simulink model "cardio_v4"  (Simulink 7.4)
settings: Solver=ode45  StartTime=0.0  StopTime=10  FixedStep=0.1  RelTol=1e-3
undefined symbols (not defined in the file): ln
(part 2 of 2)

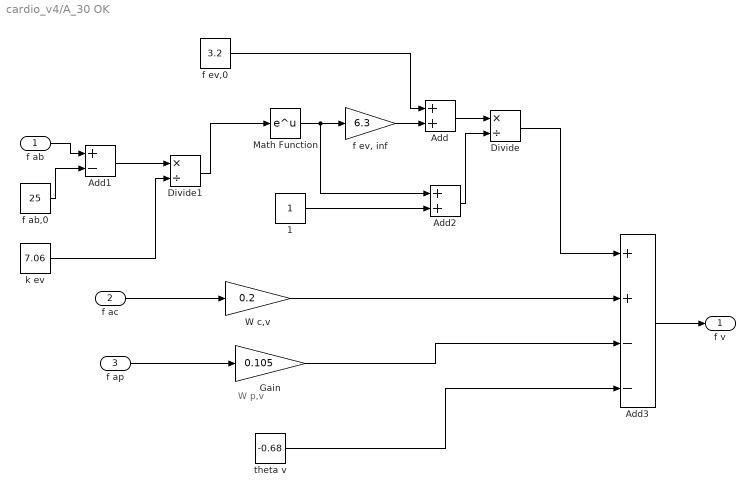
== system cardio_v4/A_30 OK ==
  note: W p,v
  f ab : Inport  OutDataType=sfix(16)  OutScaling=2^0
  f ac : Inport  Port=2  OutDataType=sfix(16)  OutScaling=2^0
  f ap : Inport  Port=3  OutDataType=sfix(16)  OutScaling=2^0
  1 : Constant  OutDataType=sfix(16)  OutScaling=2^0
  Add : Sum  OutDataType=sfix(16)  OutScaling=2^-10
  Add1 : Sum  Inputs=+-  OutDataType=sfix(16)  OutScaling=2^-10
  Add2 : Sum  OutDataType=sfix(16)  OutScaling=2^-10
  Add3 : Sum  Inputs=++--  OutDataType=sfix(16)  OutScaling=2^-10
  Divide : Product  Inputs=*/  OutDataType=sfix(16)  OutScaling=2^-10
  Divide1 : Product  Inputs=*/  OutDataType=sfix(16)  OutScaling=2^-10
  Gain : Gain  Gain=0.105  ParameterDataType=sfix(16)  ParameterScaling=2^0  OutDataType=sfix(16)  OutScaling=2^0
  Math Function : Math  OutDataType=sfix(16)  OutScaling=2^0  SaturateOnIntegerOverflow=on
  W c,v : Gain  Gain=0.2  ParameterDataType=sfix(16)  ParameterScaling=2^0  OutDataType=sfix(16)  OutScaling=2^0
  f ab,0 : Constant  Value=25  OutDataType=sfix(16)  OutScaling=2^0
  "f ev, inf" : Gain  Gain=6.3  ParameterDataType=sfix(16)  ParameterScaling=2^0  OutDataType=sfix(16)  OutScaling=2^0
  f ev,0 : Constant  Value=3.2  OutDataType=sfix(16)  OutScaling=2^0
  k ev : Constant  Value=7.06  OutDataType=sfix(16)  OutScaling=2^0
  theta v : Constant  Value=-0.68  OutDataType=sfix(16)  OutScaling=2^0
  f v : Outport  OutDataType=sfix(16)  OutScaling=2^0
  wires:
  theta v/1 -> Add3/4
  Gain/1 -> Add3/3
  f ap/1 -> Gain/1
  f ac/1 -> W c,v/1
  W c,v/1 -> Add3/2
  Add3/1 -> f v/1
  Divide/1 -> Add3/1
  1/1 -> Add2/2
  Add2/1 -> Divide/2
  k ev/1 -> Divide1/2
  Divide1/1 -> Math Function/1
  Add1/1 -> Divide1/1
  f ab,0/1 -> Add1/2
  f ab/1 -> Add1/1
  Math Function/1 -> Add2/1, "f ev, inf"/1
  "f ev, inf"/1 -> Add/2
  f ev,0/1 -> Add/1
  Add/1 -> Divide/1

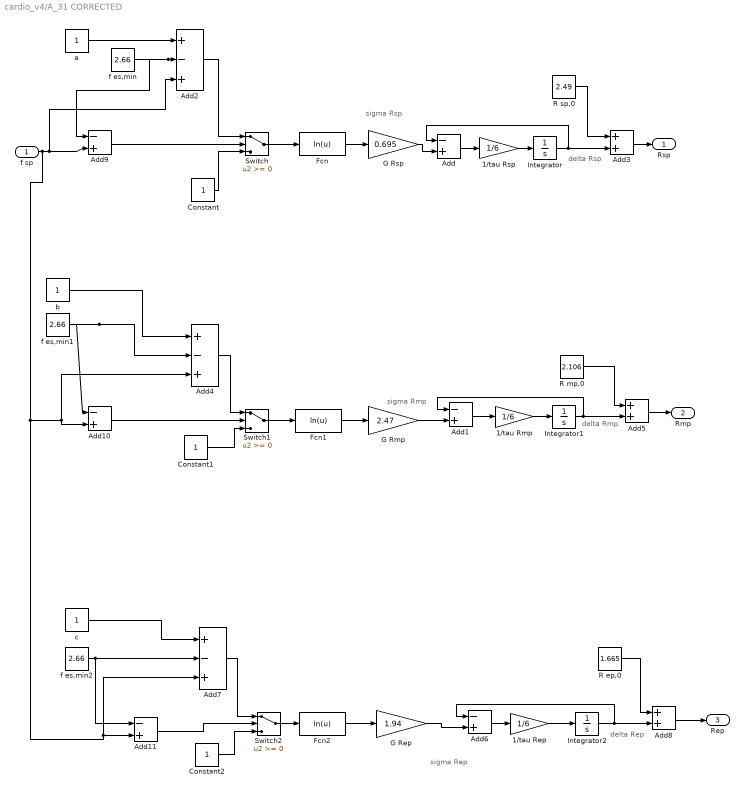
== system cardio_v4/A_31 CORRECTED ==
  note: sigma Rep
  note: delta Rep
  note: delta Rmp
  note: sigma Rmp
  note: delta Rsp
  note: sigma Rsp
  f sp : Inport  OutDataType=sfix(16)  OutScaling=2^0
  1/tau Rep : Gain  Gain=1/6  ParameterDataType=sfix(16)  ParameterScaling=2^0  OutDataType=sfix(16)  OutScaling=2^0
  1/tau Rmp : Gain  Gain=1/6  ParameterDataType=sfix(16)  ParameterScaling=2^0  OutDataType=sfix(16)  OutScaling=2^0
  1/tau Rsp : Gain  Gain=1/6  ParameterDataType=sfix(16)  ParameterScaling=2^0  OutDataType=sfix(16)  OutScaling=2^0
  Add{,1,6,9..11} (6 alike) : Sum  Inputs=-+  OutDataType=sfix(16)  OutScaling=2^-10
  Add2 : Sum  Inputs=+-+  OutDataType=sfix(16)  OutScaling=2^-10
  Add3 : Sum  OutDataType=sfix(16)  OutScaling=2^-10
  Add4 : Sum  Inputs=+-+  OutDataType=sfix(16)  OutScaling=2^-10
  Add5 : Sum  OutDataType=sfix(16)  OutScaling=2^-10
  Add7 : Sum  Inputs=+-+  OutDataType=sfix(16)  OutScaling=2^-10
  Add8 : Sum  OutDataType=sfix(16)  OutScaling=2^-10
  Constant : Constant  OutDataType=sfix(16)  OutScaling=2^0
  Constant1 : Constant  OutDataType=sfix(16)  OutScaling=2^0
  Constant2 : Constant  OutDataType=sfix(16)  OutScaling=2^0
  Fcn : Fcn  Expr=ln(u)
  Fcn1 : Fcn  Expr=ln(u)
  Fcn2 : Fcn  Expr=ln(u)
  G Rep : Gain  Gain=1.94  ParameterDataType=sfix(16)  ParameterScaling=2^0  OutDataType=sfix(16)  OutScaling=2^0
  G Rmp : Gain  Gain=2.47  ParameterDataType=sfix(16)  ParameterScaling=2^0  OutDataType=sfix(16)  OutScaling=2^0
  G Rsp : Gain  Gain=0.695  ParameterDataType=sfix(16)  ParameterScaling=2^0  OutDataType=sfix(16)  OutScaling=2^0
  Integrator : Integrator
  Integrator1 : Integrator
  Integrator2 : Integrator
  R ep,0 : Constant  Value=1.665  OutDataType=sfix(16)  OutScaling=2^0
  R mp,0 : Constant  Value=2.106  OutDataType=sfix(16)  OutScaling=2^0
  R sp,0 : Constant  Value=2.49  OutDataType=sfix(16)  OutScaling=2^0
  Switch : Switch
  Switch1 : Switch
  Switch2 : Switch
  a : Constant  OutDataType=sfix(16)  OutScaling=2^0
  b : Constant  OutDataType=sfix(16)  OutScaling=2^0
  c : Constant  OutDataType=sfix(16)  OutScaling=2^0
  f es,min : Constant  Value=2.66  OutDataType=sfix(16)  OutScaling=2^0
  f es,min1 : Constant  Value=2.66  OutDataType=sfix(16)  OutScaling=2^0
  f es,min2 : Constant  Value=2.66  OutDataType=sfix(16)  OutScaling=2^0
  Rsp : Outport  OutDataType=sfix(16)  OutScaling=2^0
  Rmp : Outport  Port=2  OutDataType=sfix(16)  OutScaling=2^0
  Rep : Outport  Port=3  OutDataType=sfix(16)  OutScaling=2^0
  wires:
  R mp,0/1 -> Add5/1
  Add5/1 -> Rmp/1
  f es,min/1 -> Add2/2, Add9/1
  a/1 -> Add2/1
  R sp,0/1 -> Add3/1
  R ep,0/1 -> Add8/1
  Add8/1 -> Rep/1
  f es,min2/1 -> Add7/2, Add11/1
  c/1 -> Add7/1
  Fcn2/1 -> G Rep/1
  Integrator2/1 -> Add8/2, Add6/1
  Add6/1 -> 1/tau Rep/1
  1/tau Rep/1 -> Integrator2/1
  f es,min1/1 -> Add4/2, Add10/1
  b/1 -> Add4/1
  Fcn1/1 -> G Rmp/1
  Integrator1/1 -> Add5/2, Add1/1
  Add1/1 -> 1/tau Rmp/1
  1/tau Rmp/1 -> Integrator1/1
  Add3/1 -> Rsp/1
  Fcn/1 -> G Rsp/1
  f sp/1 -> Add10/2, Add4/3, Add11/2, Add7/3, Add9/2, Add2/3
  Integrator/1 -> Add3/2, Add/1
  Add/1 -> 1/tau Rsp/1
  1/tau Rsp/1 -> Integrator/1
  Constant/1 -> Switch/3
  Add9/1 -> Switch/2
  Add2/1 -> Switch/1
  Switch/1 -> Fcn/1
  G Rsp/1 -> Add/2
  Add10/1 -> Switch1/2
  Constant1/1 -> Switch1/3
  Add4/1 -> Switch1/1
  Switch1/1 -> Fcn1/1
  G Rmp/1 -> Add1/2
  Constant2/1 -> Switch2/3
  Add11/1 -> Switch2/2
  Add7/1 -> Switch2/1
  Switch2/1 -> Fcn2/1
  G Rep/1 -> Add6/2

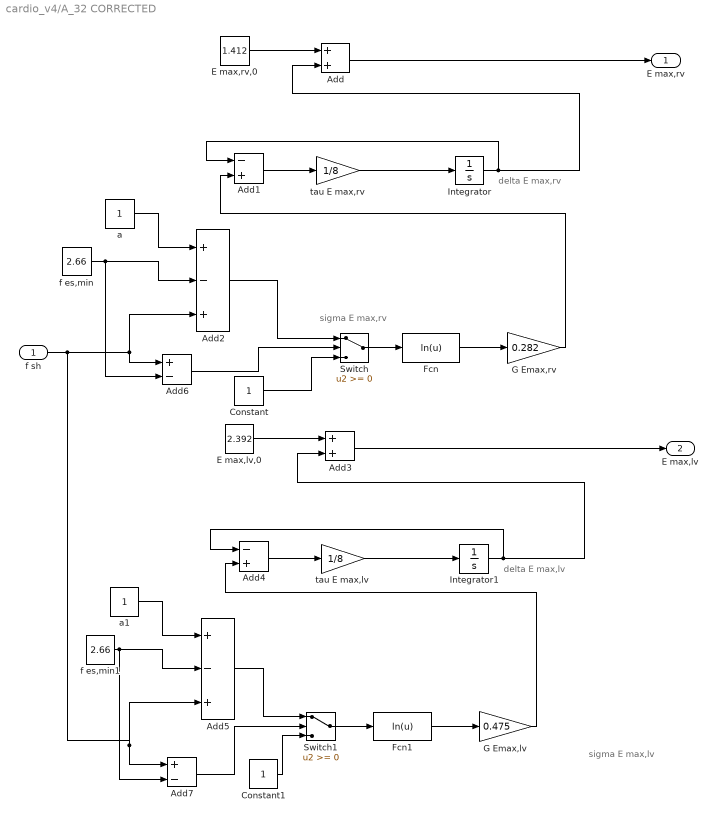
== system cardio_v4/A_32 CORRECTED ==
  note: sigma E max,lv
  note: delta E max,lv
  note: sigma E max,rv
  note: delta E max,rv
  f sh : Inport  OutDataType=sfix(16)  OutScaling=2^0
  Add : Sum  OutDataType=sfix(16)  OutScaling=2^-10
  Add1 : Sum  Inputs=-+  OutDataType=sfix(16)  OutScaling=2^-10
  Add2 : Sum  Inputs=+-+  OutDataType=sfix(16)  OutScaling=2^-10
  Add3 : Sum  OutDataType=sfix(16)  OutScaling=2^-10
  Add4 : Sum  Inputs=-+  OutDataType=sfix(16)  OutScaling=2^-10
  Add5 : Sum  Inputs=+-+  OutDataType=sfix(16)  OutScaling=2^-10
  Add6 : Sum  Inputs=+-  OutDataType=sfix(16)  OutScaling=2^-10
  Add7 : Sum  Inputs=+-  OutDataType=sfix(16)  OutScaling=2^-10
  Constant : Constant  OutDataType=sfix(16)  OutScaling=2^0
  Constant1 : Constant  OutDataType=sfix(16)  OutScaling=2^0
  E max,lv,0 : Constant  Value=2.392  OutDataType=sfix(16)  OutScaling=2^0
  E max,rv,0 : Constant  Value=1.412  OutDataType=sfix(16)  OutScaling=2^0
  Fcn : Fcn  Expr=ln(u)
  Fcn1 : Fcn  Expr=ln(u)
  G Emax,lv : Gain  Gain=0.475  ParameterDataType=sfix(16)  ParameterScaling=2^0  OutDataType=sfix(16)  OutScaling=2^0
  G Emax,rv : Gain  Gain=0.282  ParameterDataType=sfix(16)  ParameterScaling=2^0  OutDataType=sfix(16)  OutScaling=2^0
  Integrator : Integrator
  Integrator1 : Integrator
  Switch : Switch
  Switch1 : Switch
  a : Constant  OutDataType=sfix(16)  OutScaling=2^0
  a1 : Constant  OutDataType=sfix(16)  OutScaling=2^0
  f es,min : Constant  Value=2.66  OutDataType=sfix(16)  OutScaling=2^0
  f es,min1 : Constant  Value=2.66  OutDataType=sfix(16)  OutScaling=2^0
  tau E max,lv : Gain  Gain=1/8  ParameterDataType=sfix(16)  ParameterScaling=2^0  OutDataType=sfix(16)  OutScaling=2^0
  tau E max,rv : Gain  Gain=1/8  ParameterDataType=sfix(16)  ParameterScaling=2^0  OutDataType=sfix(16)  OutScaling=2^0
  E max,rv : Outport  OutDataType=sfix(16)  OutScaling=2^0
  E max,lv : Outport  Port=2  OutDataType=sfix(16)  OutScaling=2^0
  wires:
  a1/1 -> Add5/1
  f es,min1/1 -> Add5/2, Add7/2
  Fcn1/1 -> G Emax,lv/1
  Add4/1 -> tau E max,lv/1
  tau E max,lv/1 -> Integrator1/1
  Integrator1/1 -> Add3/2, Add4/1
  E max,lv,0/1 -> Add3/1
  Add3/1 -> E max,lv/1
  a/1 -> Add2/1
  f es,min/1 -> Add2/2, Add6/2
  Fcn/1 -> G Emax,rv/1
  Constant/1 -> Switch/3
  f sh/1 -> Add7/1, Add5/3, Add6/1, Add2/3
  Add1/1 -> tau E max,rv/1
  tau E max,rv/1 -> Integrator/1
  Integrator/1 -> Add/2, Add1/1
  E max,rv,0/1 -> Add/1
  Add/1 -> E max,rv/1
  Add6/1 -> Switch/2
  Add2/1 -> Switch/1
  Switch/1 -> Fcn/1
  G Emax,rv/1 -> Add1/2
  Constant1/1 -> Switch1/3
  Add7/1 -> Switch1/2
  Add5/1 -> Switch1/1
  Switch1/1 -> Fcn1/1
  G Emax,lv/1 -> Add4/2

== system cardio_v4/A1_19 CORRECTED/beta(H) ==
  H : Inport  OutDataType=sfix(16)  OutScaling=2^0
  alpha : Inport  Port=2  OutDataType=sfix(16)  OutScaling=2^0
  n : Inport  Port=3  OutDataType=sfix(16)  OutScaling=2^0
  m : Inport  Port=4  OutDataType=sfix(16)  OutScaling=2^0
  Add : Sum  OutDataType=sfix(16)  OutScaling=2^-10
  Add1 : Sum  Inputs=+-  OutDataType=sfix(16)  OutScaling=2^-10
  Divide : Product  Inputs=**/  OutDataType=sfix(16)  OutScaling=2^-10
  Product : Product  OutDataType=sfix(16)  OutScaling=2^0  RndMeth=Zero
  t p(H) : Fcn  Expr=0.1859+(1/(u^9.9+1))*(0.2799-0.1859)
  Out1 : Outport  OutDataType=sfix(16)  OutScaling=2^0
  wires:
  n/1 -> Add/1, Divide/3
  m/1 -> Add/2, Divide/2
  Add/1 -> Product/2
  t p(H)/1 -> Product/1
  H/1 -> t p(H)/1
  Product/1 -> Add1/1
  alpha/1 -> Divide/1
  Divide/1 -> Add1/2
  Add1/1 -> Out1/1

== matlab function A1_19 CORRECTED/Embedded MATLAB Function ==
  data: t input double; y output double; Hmin input double
function y = fcn(t,Hmin)
% This block supports an embeddable subset of the MATLAB language.
% See the help menu for details. 

y = mod(t,60/Hmin);
